simulink model "pdcontrol"  (R2013b)
settings: Solver=ode45  StartTime=0.0  StopTime=10000000000000000  RelTol=1e-3
InitFcn:
  | param
undefined symbols (not defined in the file or in its folder): AP, can_ctrl
settings Model: Creator=paul  LastModifiedBy=paul

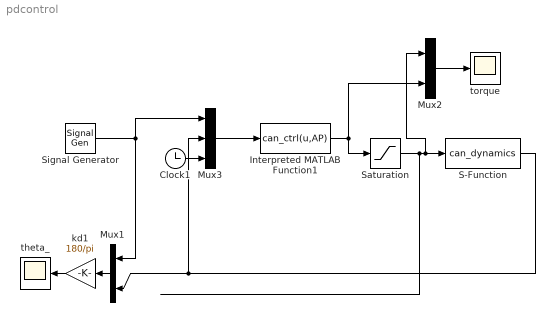
== system pdcontrol ==
  Clock1 : Clock
  Interpreted MATLAB Function1 : MATLABFcn  MATLABFcn=can_ctrl(u,AP)  OutputDimensions=1  SampleTime=AP.Ts
  Mux1 : Mux  Inputs=2
  Mux2 : Mux  Inputs=2
  Mux3 : Mux  Inputs=3
  S-Function : S-Function  FunctionName=can_dynamics  Parameters=AP  EnableBusSupport=off
  Saturation : Saturate  UpperLimit=AP.F_max  LowerLimit=-AP.F_max  SampleTime=AP.Ts
  Signal Generator : SignalGenerator  Amplitude=pi/4
  kd1 : Gain  Gain=180/pi
  theta_ : Scope
      settings: TimeRange=10  YMin=-65  YMax=50
  torque : Scope
      settings: TimeRange=10  YMin=-1  YMax=7
  wires:
  Signal Generator/1 -> Mux1/1, Mux3/1
  kd1/1 -> theta_/1
  Mux1/1 -> kd1/1
  Interpreted MATLAB Function1/1 -> Mux2/2, Saturation/1
  Mux2/1 -> torque/1
  Saturation/1 -> Mux2/1, S-Function/1
  Mux3/1 -> Interpreted MATLAB Function1/1
  Clock1/1 -> Mux3/3
  S-Function/1 -> Mux1/2, Mux3/2
